simulink model "Dynamics_2024"  (R2024b)
settings: Solver=FixedStepAuto  StartTime=0  StopTime=268704.3823  FixedStep=10  RelTol=1e-12  AbsTol=1e-12
values from neighbouring files (symbols this model uses):
  Disturbances = 1    [Main.m]
  kd = 1e-3    (= 0.001)    [Main.m]
  ki = 1e-3    (= 0.001)    [Main.m]
  kp = 2    [Main.m]
  q0 = [  -0.197305854517669 ... (first row only)    [Main.m]
undefined symbols (not defined in the file or in its folder): control, epsilon, Fe_sun, G, Ix, Iy, Iz, J_e, magnitude, mt, mu_e, mu_sun, r_0ts, R_e, Satellite, v0, v_0ts, w_0, w_desired, x0
libraries: matrix_library x2, vrlib x1
settings Model: Creator=marty  LastModifiedBy=marty

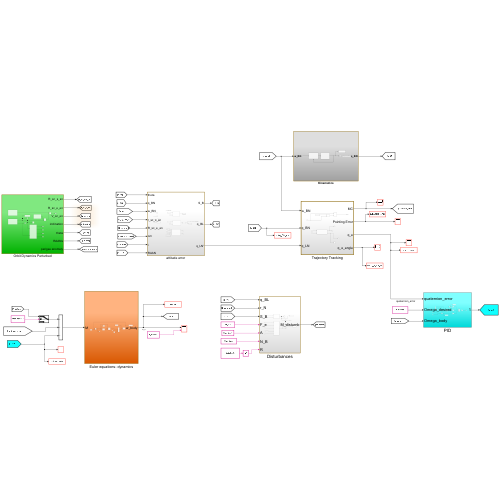
[thumbnail: Simulink's stored preview of the top-level diagram]
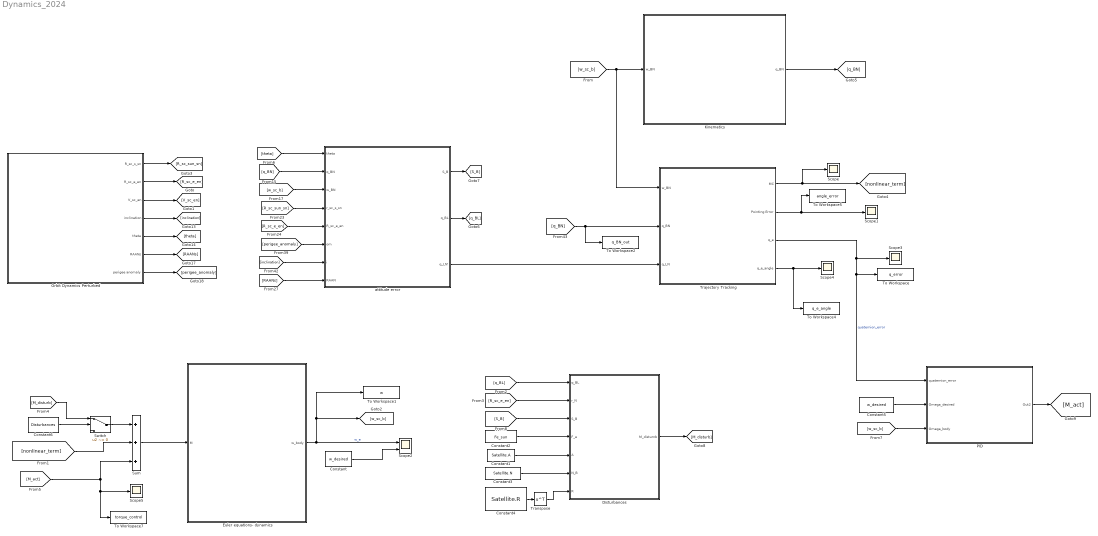
== system Dynamics_2024 ==
  Constant : Constant  Value=w_desired
  Constant1 : Constant  Value=Satellite.A
  Constant2 : Constant  Value=Fe_sun
  Constant3 : Constant  Value=Satellite.N
  Constant4 : Constant  Value=Satellite.R
  Constant5 : Constant  Value=w_desired
  Constant6 : Constant  Value=Disturbances
  Disturbances : Subsystem
  Euler equations- dynamics : Subsystem
  Kinematics : Subsystem
  Orbit Dynamics Perturbed : Subsystem
  PID : Subsystem
  Scope{,1,3..5} (5 alike) : Scope
  Scope2 : Scope  NumInputPorts=2
  Sum : Sum  Inputs=+++
  Switch : Switch  Criteria=u2 ~= 0  SaturateOnIntegerOverflow=off  InputSameDT=off
  To Workspace : ToWorkspace  VariableName=q_error  SampleTime=-1
  To Workspace1 : ToWorkspace  VariableName=w  SampleTime=-1
  To Workspace2 : ToWorkspace  VariableName=q_BN_out  SampleTime=-1
  To Workspace4 : ToWorkspace  VariableName=q_e_angle  SampleTime=-1
  To Workspace5 : ToWorkspace  VariableName=angle_error  SampleTime=-1
  To Workspace7 : ToWorkspace  VariableName=torque_control  SampleTime=-1
  Trajectory Tracking : Subsystem  TreatAsAtomicUnit=on
  Transpose : Math  Operator=transpose
  attitude error : Subsystem
  wires:
  attitude error/2(q_BL) -> [q_BL]
  [R_sc_e_en] -> attitude error/5(R_sc_e_en)
  Orbit Dynamics Perturbed/7(perigee anomaly) -> [perigee_anomaly]
  Constant/1 -> Scope2/2
  [inclination] -> attitude error/7(i)
  [R_sc_sun_sn] -> attitude error/4(r_sc_s_sn)
  Trajectory Tracking/2(Pointing Error) -> To Workspace5/1, Scope1/1
  attitude error/3(q_LN') -> Trajectory Tracking/3(q_LN)
  Orbit Dynamics Perturbed/1(R_sc_s_sn) -> [R_sc_sun_sn]
  Orbit Dynamics Perturbed/2(R_sc_e_en) -> [R_sc_e_en]
  Orbit Dynamics Perturbed/4(inclination) -> [inclination]
  [w_sc_b] -> attitude error/3(w_BN)
  [w_sc_b] -> Kinematics/1(w_BN), Trajectory Tracking/1(w_BN)
  [perigee_anomaly] -> attitude error/6(om)
  Orbit Dynamics Perturbed/3(V_sc_en) -> [V_sc_en]
  Orbit Dynamics Perturbed/6(RAANs) -> [RAANs]
  Sum/1 -> Euler equations- dynamics/1(M)
  [RAANs] -> attitude error/8(RAAN)
  [q_BN] -> attitude error/2(q_BN)
  attitude error/1(S_B) -> [S_B]
  Kinematics/1(q_BN) -> [q_BN]
  Orbit Dynamics Perturbed/5(theta) -> [theta]
  [theta] -> attitude error/1(theta)
  [q_BN] -> To Workspace2/1, Trajectory Tracking/2(q_BN)
  Constant4/1 -> Transpose/1
  [q_BL] -> Disturbances/1(q_BL)
  [R_sc_e_en] -> Disturbances/2(r_N)
  [S_B] -> Disturbances/3(S_B)
  Constant2/1 -> Disturbances/4(F_e)
  Constant1/1 -> Disturbances/5(A)
  Constant3/1 -> Disturbances/6(N_B)
  Transpose/1 -> Disturbances/7(R)
  Disturbances/1(M_disturnb) -> [M_disturb]
  [M_disturb] -> Switch/1
  Trajectory Tracking/4(q_e_angle) -> To Workspace4/1, Scope4/1
  Euler equations- dynamics/1(w_body) -> To Workspace1/1, [w_sc_b], Scope2/1  "w_e"
  Trajectory Tracking/3(q_e) -> PID/1(quaternion_error), To Workspace/1, Scope3/1  "quaternion_error"
  Trajectory Tracking/1(MC) -> Scope/1, [nonlinear_term]
  [nonlinear_term] -> Sum/2
  Switch/1 -> Sum/1
  Constant6/1 -> Switch/2
  [M_act] -> Sum/3, Scope5/1, To Workspace7/1
  Constant5/1 -> PID/2(Omega_desired)
  [w_sc_b] -> PID/3(Omega_body)
  PID/1(Out2) -> [M_act]

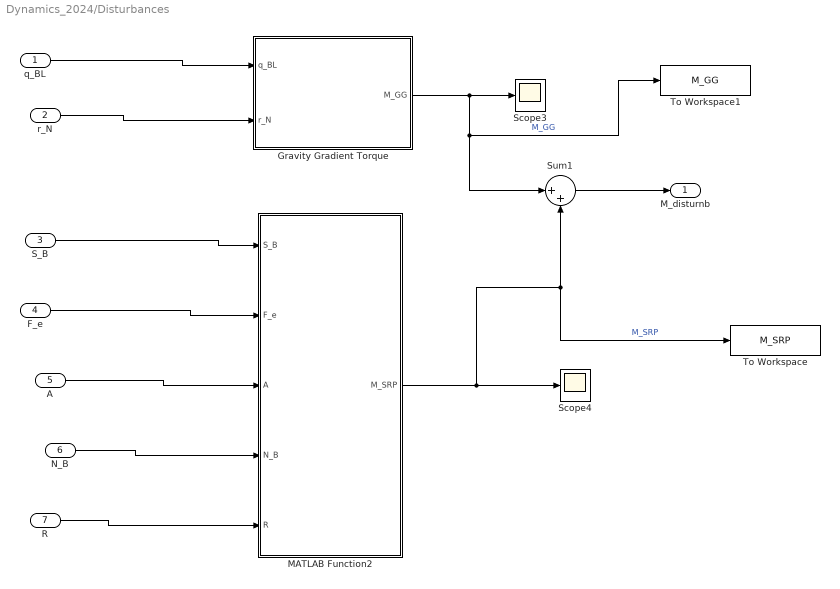
== system Dynamics_2024/Disturbances ==
  q_BL : Inport
  r_N : Inport  Port=2
  S_B : Inport  Port=3
  F_e : Inport  Port=4
  A : Inport  Port=5
  N_B : Inport  Port=6
  R : Inport  Port=7
  Gravity Gradient Torque : Subsystem
  MATLAB Function2 : MATLAB Function  TreatAsAtomicUnit=on
  Scope3 : Scope
  Scope4 : Scope
  Sum1 : Sum  Inputs=|++
  To Workspace : ToWorkspace  VariableName=M_SRP  SampleTime=-1
  To Workspace1 : ToWorkspace  VariableName=M_GG  SampleTime=-1
  M_disturnb : Outport
  wires:
  R/1 -> MATLAB Function2/5(R)
  MATLAB Function2/1(M_SRP) -> Sum1/2, To Workspace/1, Scope4/1  "M_SRP"
  F_e/1 -> MATLAB Function2/2(F_e)
  Gravity Gradient Torque/1(M_GG) -> To Workspace1/1, Sum1/1, Scope3/1  "M_GG"
  q_BL/1 -> Gravity Gradient Torque/1(q_BL)
  r_N/1 -> Gravity Gradient Torque/2(r_N)
  N_B/1 -> MATLAB Function2/4(N_B)
  A/1 -> MATLAB Function2/3(A)
  S_B/1 -> MATLAB Function2/1(S_B)
  Sum1/1 -> M_disturnb/1

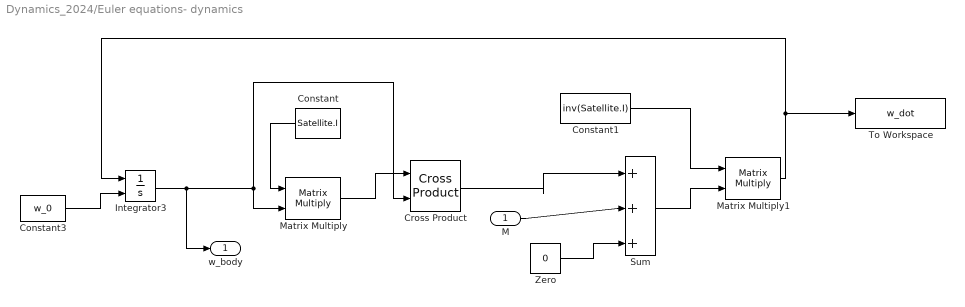
== system Dynamics_2024/Euler equations- dynamics ==
  M : Inport
  Constant : Constant  Value=Satellite.I
  Constant1 : Constant  Value=inv(Satellite.I)
  Constant3 : Constant  Value=w_0
  Cross Product : matrix_library/Cross Product
  Integrator3 : Integrator  InitialConditionSource=external
  Matrix Multiply : Product  Multiplication=Matrix(*)
  Matrix Multiply1 : Product  Multiplication=Matrix(*)
  Sum : Sum  Inputs=|+++
  To Workspace : ToWorkspace  VariableName=w_dot  SampleTime=-1
  Zero : Constant  Value=0  OutDataTypeStr=Inherit: Inherit via back propagation
  w_body : Outport
  wires:
  Constant3/1 -> Integrator3/2
  Integrator3/1 -> w_body/1, Matrix Multiply/2, Cross Product/2
  Matrix Multiply/1 -> Cross Product/1
  Constant1/1 -> Matrix Multiply1/1
  Matrix Multiply1/1 -> Integrator3/1, To Workspace/1
  Constant/1 -> Matrix Multiply/1
  Cross Product/1 -> Sum/1
  Sum/1 -> Matrix Multiply1/2
  M/1 -> Sum/2
  Zero/1 -> Sum/3

== system Dynamics_2024/Kinematics ==
  note: (Body Frame Quaternion)
  w_BN : Inport
  Quaternion Normalisation : Subsystem
  Quaternions : Subsystem
      settings: PortSchema="{\"entries\":[{\"content\":{\"sides\":[{\"content\":{\"connectorIds\":[\"In1\"]},\"type\":\"ConnectorPlacement.EquallySpacedRectSide\",\"uuid\":\"337480c7-b996-434a-97d1-93b75d8b293c\"},{\"content\":{\"connectorIds\":[\"Out1\"],\"side\":\"RIGHT\"},\"type\":\"ConnectorPlacement.EquallySpacedRectSide\",\"uuid\":\"41d32615-4344-48a4-ad5b-2dad4deabdda\"},{\"content\":{\"side\":\"TOP\"},\"type\":\"ConnectorPlacement.EquallySpacedRectSide\",\"uuid\":\"47835596-097d-48d1-90ae-77b48fddf76d\"},{\"content\":{\"connectorIds\":[\"In2\"],\"side\":\"BOTTOM\"},\"type\":\"ConnectorPlacement.EquallySpacedRectSide\",\"uuid\":\"9f38fa4d-c6c1-4321-9750-02b4f73c744f\"}]},\"type\":\"ConnectorPlacement.EquallySpacedConnector\",\"uuid\":\"8ea16f6d-57f4-43cd-ae9c-44a64026dd8f\"}],\"packageUris\":[\"http://schema.mathworks.com/mf0/Connector/R2020b\"],\"version\":\"1.0\"}"
  To Workspace : ToWorkspace  VariableName=q_BN  SampleTime=-1
  q_BN : Outport
  wires:
  w_BN/1 -> Quaternions/1(w)
  Quaternion Normalisation/1(q_BN) -> To Workspace/1, q_BN/1, Quaternions/2(q_BN)
  Quaternions/1(q(t)) -> Quaternion Normalisation/1(q(t))

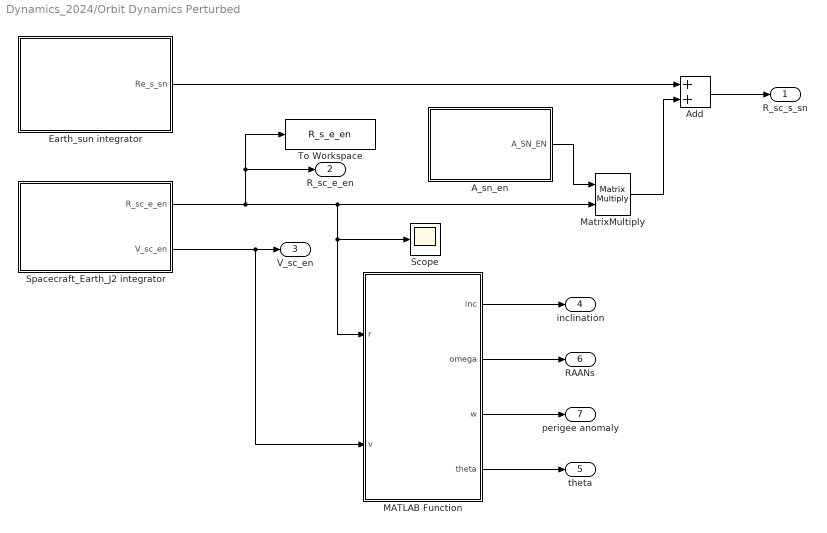
== system Dynamics_2024/Orbit Dynamics Perturbed ==
  A_sn_en : Subsystem
  Add : Sum
  Earth_sun integrator : Subsystem
  MATLAB Function : MATLAB Function  TreatAsAtomicUnit=on
  MatrixMultiply : Product  Multiplication=Matrix(*)
  Scope : Scope
  "Spacecraft_Earth_J2 integrator " : Subsystem
  To Workspace : ToWorkspace  VariableName=R_s_e_en  SampleTime=-1
  R_sc_s_sn : Outport
  R_sc_e_en : Outport  Port=2
  V_sc_en : Outport  Port=3
  inclination : Outport  Port=4
  theta : Outport  Port=5
  RAANs : Outport  Port=6
  perigee anomaly : Outport  Port=7
  wires:
  MatrixMultiply/1 -> Add/2
  A_sn_en/1(A_SN_EN) -> MatrixMultiply/1
  "Spacecraft_Earth_J2 integrator "/2(V_sc_en) -> MATLAB Function/2(v), V_sc_en/1
  "Spacecraft_Earth_J2 integrator "/1(R_sc_e_en) -> R_sc_e_en/1, To Workspace/1, Scope/1, MATLAB Function/1(r), MatrixMultiply/2
  Earth_sun integrator/1(Re_s_sn) -> Add/1
  Add/1 -> R_sc_s_sn/1
  MATLAB Function/1(inc) -> inclination/1
  MATLAB Function/4(theta) -> theta/1
  MATLAB Function/2(omega) -> RAANs/1
  MATLAB Function/3(w) -> perigee anomaly/1

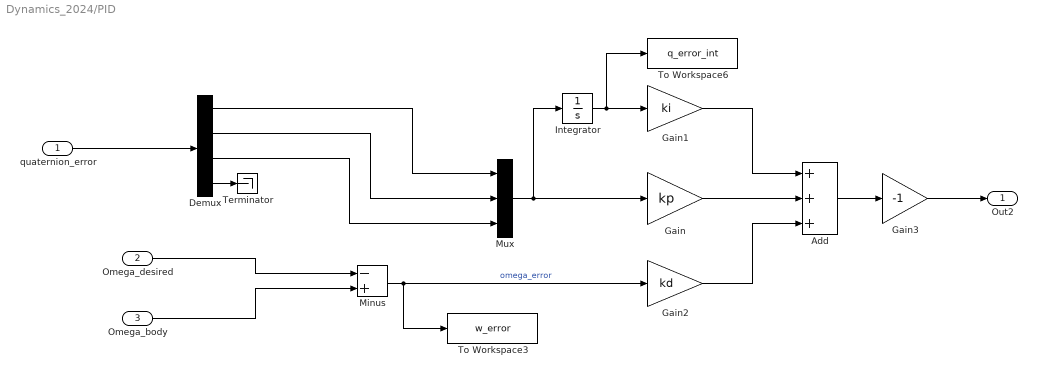
== system Dynamics_2024/PID ==
  quaternion_error : Inport
  Omega_desired : Inport  Port=2
  Omega_body : Inport  Port=3
  Add : Sum  Inputs=+++
  Demux : Demux
  Gain : Gain  Gain=kp
  Gain1 : Gain  Gain=ki
  Gain2 : Gain  Gain=kd
  Gain3 : Gain  Gain=-1
  Integrator : Integrator
  Minus : Sum  Inputs=-+
  Mux : Mux  Inputs=3
  Terminator : Terminator
  To Workspace3 : ToWorkspace  VariableName=w_error  SampleTime=-1
  To Workspace6 : ToWorkspace  VariableName=q_error_int  SampleTime=-1
  Out2 : Outport
  wires:
  Minus/1 -> To Workspace3/1, Gain2/1  "omega_error"
  Integrator/1 -> To Workspace6/1, Gain1/1
  Add/1 -> Gain3/1
  Demux/2 -> Mux/2
  Demux/3 -> Mux/3
  Gain1/1 -> Add/1
  Omega_desired/1 -> Minus/1
  Demux/1 -> Mux/1
  Gain2/1 -> Add/3
  Mux/1 -> Integrator/1, Gain/1
  Gain/1 -> Add/2
  Demux/4 -> Terminator/1
  Omega_body/1 -> Minus/2
  Gain3/1 -> Out2/1
  quaternion_error/1 -> Demux/1

== system Dynamics_2024/Trajectory Tracking ==
  note: ref
  w_BN : Inport
  q_BN : Inport  Port=2
  q_LN : Inport  Port=3
  Constant2 : Constant  Value=Satellite.I
  Cross Product : matrix_library/Cross Product
  Pointing Error for Slew Maneuvre : Subsystem
  Product1 : Product  Multiplication=Matrix(*)
  Scope : Scope
  MC : Outport
  Pointing Error : Outport  Port=2
  q_e : Outport  Port=3
  q_e_angle : Outport  Port=4
  wires:
  q_BN/1 -> Pointing Error for Slew Maneuvre/2(q_Est)  "q_BN"
  Product1/1 -> Cross Product/2
  Constant2/1 -> Product1/1
  Cross Product/1 -> MC/1
  w_BN/1 -> Product1/2, Cross Product/1
  q_LN/1 -> Pointing Error for Slew Maneuvre/1(q_LN)
  Pointing Error for Slew Maneuvre/1(Pointing Error) -> q_e_angle/1, Pointing Error/1  "pointing error"
  Pointing Error for Slew Maneuvre/2(q_e) -> Scope/1, q_e/1  "q_e"

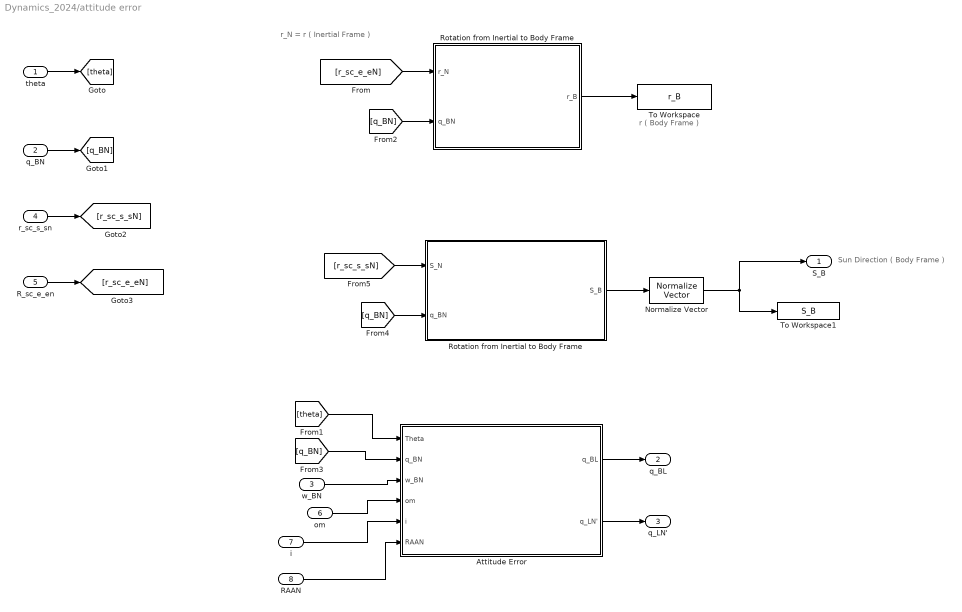
== system Dynamics_2024/attitude error ==
  note: r_N = r ( Inertial Frame )
  note: Sun Direction ( Body Frame )
  note: r ( Body Frame )
  theta : Inport
  q_BN : Inport  Port=2
  w_BN : Inport  Port=3
  r_sc_s_sn : Inport  Port=4
  R_sc_e_en : Inport  Port=5
  om : Inport  Port=6
  i : Inport  Port=7
  RAAN : Inport  Port=8
  " Rotation from Inertial to Body Frame" : Subsystem
  Attitude Error : Subsystem
  Normalize Vector : vrlib/Utilities/Normalize Vector  maxzero=0
  Rotation from Inertial to Body Frame : Subsystem
  To Workspace : ToWorkspace  VariableName=r_B  SampleTime=-1
  To Workspace1 : ToWorkspace  VariableName=S_B  SampleTime=-1
  S_B : Outport
  q_BL : Outport  Port=2
  q_LN' : Outport  Port=3
  wires:
  Normalize Vector/1 -> S_B/1, To Workspace1/1
  w_BN/1 -> Attitude Error/3(w_BN)
  Rotation from Inertial to Body Frame/1(S_B) -> Normalize Vector/1
  " Rotation from Inertial to Body Frame"/1(r_B) -> To Workspace/1
  Attitude Error/1(q_BL) -> q_BL/1
  Attitude Error/2(q_LN') -> q_LN'/1
  theta/1 -> [theta]
  [theta] -> Attitude Error/1(Theta)
  q_BN/1 -> [q_BN]
  [q_BN] -> " Rotation from Inertial to Body Frame"/2(q_BN)
  [q_BN] -> Attitude Error/2(q_BN)
  [q_BN] -> Rotation from Inertial to Body Frame/2(q_BN)
  r_sc_s_sn/1 -> [r_sc_s_sN]
  [r_sc_e_eN] -> " Rotation from Inertial to Body Frame"/1(r_N)
  R_sc_e_en/1 -> [r_sc_e_eN]
  [r_sc_s_sN] -> Rotation from Inertial to Body Frame/1(S_N)
  om/1 -> Attitude Error/4(om)
  i/1 -> Attitude Error/5(i)
  RAAN/1 -> Attitude Error/6(RAAN)

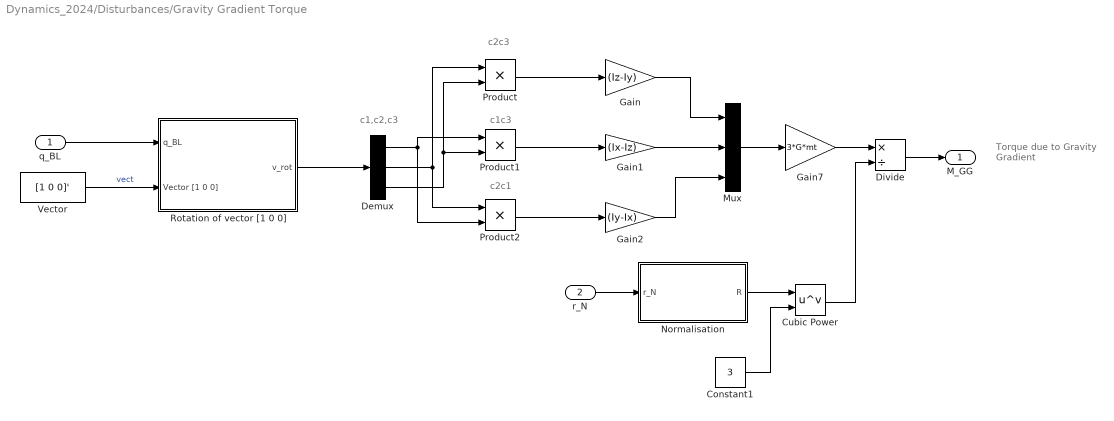
== system Dynamics_2024/Disturbances/Gravity Gradient Torque ==
  note: Torque due to
      | Gravity Gradient
  note: c1c3
  note: c2c3
  note: c2c1
  note: c1,c2,c3
  q_BL : Inport
  r_N : Inport  Port=2
  Constant1 : Constant  Value=3
  Cubic Power : Math  Operator=pow
  Demux : Demux  Outputs=3
  Divide : Product  Inputs=*/
  Gain : Gain  Gain=(Iz-Iy)
  Gain1 : Gain  Gain=(Ix-Iz)
  Gain2 : Gain  Gain=(Iy-Ix)
  Gain7 : Gain  Gain=3*G*mt
  Mux : Mux  Inputs=3
  Normalisation : Subsystem
  Product : Product
  Product1 : Product
  Product2 : Product
  Rotation of vector [1 0 0] : Subsystem
  Vector : Constant  Value=[1 0 0]'
  M_GG : Outport
  wires:
  Cubic Power/1 -> Divide/2
  Demux/1 -> Product1/1, Product2/2
  q_BL/1 -> Rotation of vector [1 0 0]/1(q_BL)
  Rotation of vector [1 0 0]/1(v_rot) -> Demux/1
  Normalisation/1(R) -> Cubic Power/1
  Divide/1 -> M_GG/1
  Vector/1 -> Rotation of vector [1 0 0]/2(Vector [1 0 0])  "vect"
  Product2/1 -> Gain2/1
  Demux/2 -> Product/1, Product2/1
  Mux/1 -> Gain7/1
  r_N/1 -> Normalisation/1(r_N)
  Gain7/1 -> Divide/1
  Demux/3 -> Product1/2, Product/2
  Constant1/1 -> Cubic Power/2
  Gain/1 -> Mux/1
  Gain1/1 -> Mux/2
  Gain2/1 -> Mux/3
  Product1/1 -> Gain1/1
  Product/1 -> Gain/1

== system Dynamics_2024/Kinematics/Quaternion Normalisation ==
  q(t) : Inport
  Divide : Product  Inputs=*/
  Dot Product : DotProduct  OutDataTypeStr=Inherit: Inherit via internal rule
  Sqrt : Sqrt
  q_BN : Outport
  wires:
  Dot Product/1 -> Sqrt/1
  q(t)/1 -> Divide/1, Dot Product/1, Dot Product/2
  Sqrt/1 -> Divide/2
  Divide/1 -> q_BN/1

== system Dynamics_2024/Kinematics/Quaternions ==
  note: Normalised
      | quaternion
  w : Inport
  q_BN : Inport  Port=2
  Gain : Gain  Gain=1/2
  Initial Condition : Constant  Value=q0
  Integrator : Integrator  InitialConditionSource=external
  Matrix Multiply : Product  Multiplication=Matrix(*)
  OMEGA Matrix : Subsystem
  q(t) : Outport
  wires:
  Integrator/1 -> q(t)/1
  Initial Condition/1 -> Integrator/2
  Matrix Multiply/1 -> Integrator/1
  Gain/1 -> Matrix Multiply/1
  w/1 -> OMEGA Matrix/1(w)
  OMEGA Matrix/1(OM Matrix) -> Gain/1
  q_BN/1 -> Matrix Multiply/2

== system Dynamics_2024/Orbit Dynamics Perturbed/A_sn_en ==
  Constant : Constant  Value=epsilon
  Constant1 : Constant
  Gain : Gain  Gain=-1
  Matrix Concatenate : Concatenate  NumInputs=3  Mode=Multidimensional array  ConcatenateDimension=2
  Mux : Mux  Inputs=3
  Mux1 : Mux  Inputs=3
  Mux2 : Mux  Inputs=3
  Trigonometric Function : Trigonometry
  Trigonometric Function1 : Trigonometry  Operator=cos
  Zero : Constant  Value=0  OutDataTypeStr=Inherit: Inherit via back propagation
  A_SN_EN : Outport
  wires:
  Gain/1 -> Mux2/3
  Constant/1 -> Trigonometric Function/1, Trigonometric Function1/1
  Trigonometric Function/1 -> Mux1/2, Gain/1
  Trigonometric Function1/1 -> Mux2/2, Mux1/3
  Constant1/1 -> Mux/1
  Mux1/1 -> Matrix Concatenate/3
  Mux/1 -> Matrix Concatenate/1
  Matrix Concatenate/1 -> A_SN_EN/1
  Mux2/1 -> Matrix Concatenate/2
  Zero/1 -> Mux/2, Mux/3, Mux2/1, Mux1/1

== system Dynamics_2024/Orbit Dynamics Perturbed/Earth_sun integrator ==
  Constant1 : Constant  Value=v_0ts
  Constant3 : Constant  Value=r_0ts
  Constant5 : Constant  Value=3
  Divide : Product  Inputs=*/
  Gain : Gain  Gain=-mu_sun
  Integrator : Integrator  InitialConditionSource=external
  Integrator1 : Integrator  InitialConditionSource=external
  Power : Math  Operator=pow
  norm : Subsystem
  Re_s_sn : Outport
  wires:
  Constant1/1 -> Integrator/2
  Constant3/1 -> Integrator1/2
  Integrator1/1 -> norm/1(vector), Divide/1, Re_s_sn/1
  Gain/1 -> Integrator/1
  Power/1 -> Divide/2
  norm/1(norm(vector)) -> Power/1
  Constant5/1 -> Power/2
  Integrator/1 -> Integrator1/1
  Divide/1 -> Gain/1

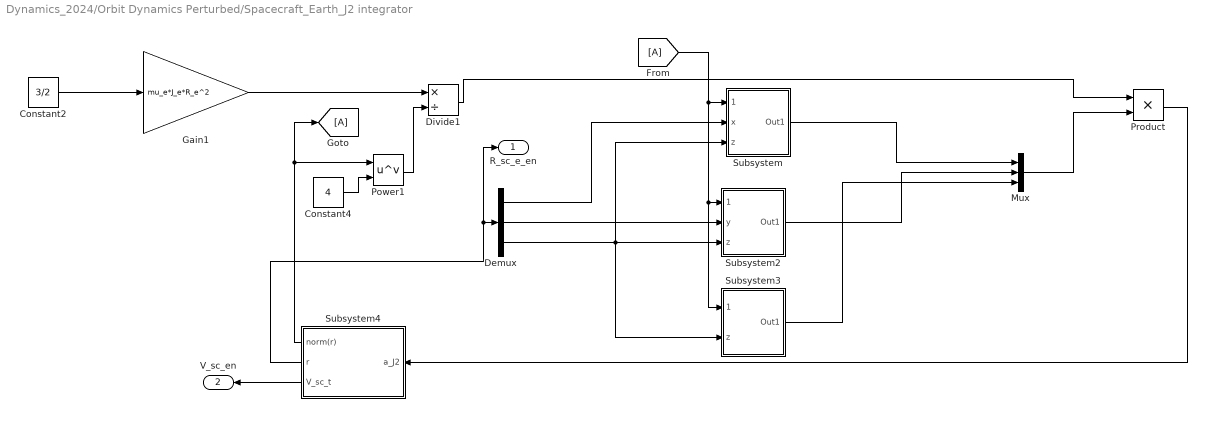
== system Dynamics_2024/Orbit Dynamics Perturbed/Spacecraft_Earth_J2 integrator  ==
  Constant2 : Constant  Value=3/2
  Constant4 : Constant  Value=4
  Demux : Demux  Outputs=3
  Divide1 : Product  Inputs=*/
  From : From
  Gain1 : Gain  Gain=mu_e*J_e*R_e^2
  Goto : Goto
  Mux : Mux  Inputs=3
  Power1 : Math  Operator=pow
  Product : Product
  Subsystem : Subsystem
  Subsystem2 : Subsystem
  Subsystem3 : Subsystem
  Subsystem4 : Subsystem
  R_sc_e_en : Outport
  V_sc_en : Outport  Port=2
  wires:
  Subsystem4/3(V_sc_t) -> V_sc_en/1
  Subsystem4/1(norm(r)) -> Power1/1, Goto/1
  Constant4/1 -> Power1/2
  Demux/2 -> Subsystem2/2(y)
  Divide1/1 -> Product/1
  From/1 -> Subsystem/1(norm(r)), Subsystem2/1(norm(r)), Subsystem3/1(norm(r))
  Demux/3 -> Subsystem3/2(z), Subsystem/3(z), Subsystem2/3(z)
  Constant2/1 -> Gain1/1
  Subsystem3/1(Out1) -> Mux/3
  Subsystem2/1(Out1) -> Mux/2
  Subsystem/1(Out1) -> Mux/1
  Product/1 -> Subsystem4/1(a_J2)
  Demux/1 -> Subsystem/2(x)
  Power1/1 -> Divide1/2
  Gain1/1 -> Divide1/1
  Subsystem4/2(r) -> Demux/1, R_sc_e_en/1
  Mux/1 -> Product/2

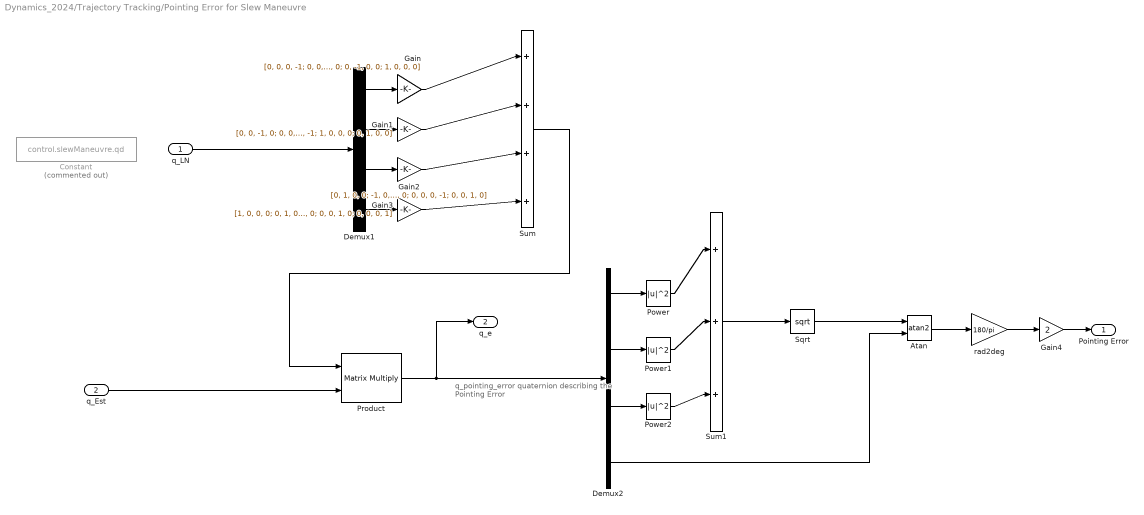
== system Dynamics_2024/Trajectory Tracking/Pointing Error for Slew Maneuvre ==
  note: q_pointing_error
      | quaternion describing the Pointing Error
  q_LN : Inport
  q_Est : Inport  Port=2
  Atan : Trigonometry  Operator=atan2  OutputSignalType=real
  Constant : Constant  Commented=on  Value=control.slewManeuvre.qd
  Demux1 : Demux
  Demux2 : Demux
  Gain : Gain  Gain=[0, 0, 0, -1; 0, 0, 1, 0; 0, -1, 0, 0; 1, 0, 0, 0]
  Gain1 : Gain  Gain=[0, 0, -1, 0; 0, 0, 0, -1; 1, 0, 0, 0; 0, 1, 0, 0]
  Gain2 : Gain  Gain=[0, 1, 0, 0; -1, 0, 0, 0; 0, 0, 0, -1; 0, 0, 1, 0]
  Gain3 : Gain  Gain=[1, 0, 0, 0; 0, 1, 0, 0; 0, 0, 1, 0; 0, 0, 0, 1]
  Gain4 : Gain  Gain=2
  Power : Math  Operator=magnitude^2
  Power1 : Math  Operator=magnitude^2
  Power2 : Math  Operator=magnitude^2
  Product : Product  Multiplication=Matrix(*)
  Sqrt : Sqrt
  Sum : Sum  Inputs=|++++
  Sum1 : Sum  Inputs=|+++
  rad2deg : Gain  Gain=180/pi
  Pointing Error : Outport
  q_e : Outport  Port=2
  wires:
  Power1/1 -> Sum1/2
  Demux2/4 -> Atan/2
  Atan/1 -> rad2deg/1
  Power/1 -> Sum1/1
  Demux2/2 -> Power1/1
  Demux2/3 -> Power2/1
  Demux2/1 -> Power/1
  Sum1/1 -> Sqrt/1
  Power2/1 -> Sum1/3
  Sqrt/1 -> Atan/1
  Product/1 -> Demux2/1, q_e/1
  Gain/1 -> Sum/1
  Gain2/1 -> Sum/3
  Gain1/1 -> Sum/2
  Demux1/3 -> Gain2/1
  Demux1/1 -> Gain/1
  Gain3/1 -> Sum/4
  Demux1/2 -> Gain1/1
  Demux1/4 -> Gain3/1
  Sum/1 -> Product/1
  rad2deg/1 -> Gain4/1
  q_LN/1 -> Demux1/1
  Gain4/1 -> Pointing Error/1
  q_Est/1 -> Product/2

== system Dynamics_2024/attitude error/ Rotation from Inertial to Body Frame ==
  note: Quaternion Rotation (Double Tensor Product)
  note: $r_B = q_{BN}\cdot r_N$
  r_N : Inport
  q_BN : Inport  Port=2
  Demux : Demux
  Mux : Mux  Inputs=3
  Quaternion multiplication 1 : Subsystem
  Quaternion multiplication 2 : Subsystem
  Transformation in Quaternion : Subsystem
  Transpose : Gain  Gain=[-1 -1 -1 1]
  r_B : Outport
  wires:
  r_N/1 -> Transformation in Quaternion/1(r_N)
  Mux/1 -> r_B/1
  Transpose/1 -> Quaternion multiplication 1/1(q_BN (T) = q)
  q_BN/1 -> Quaternion multiplication 2/2(q_BN = q'), Transpose/1
  Transformation in Quaternion/1(q(r_N)) -> Quaternion multiplication 1/2(q(r_N) = q')
  Quaternion multiplication 2/1(q*q' = q2) -> Demux/1
  Quaternion multiplication 1/1(q*q' = q1) -> Quaternion multiplication 2/1(q1 = q)
  Demux/1 -> Mux/1
  Demux/2 -> Mux/2
  Demux/3 -> Mux/3

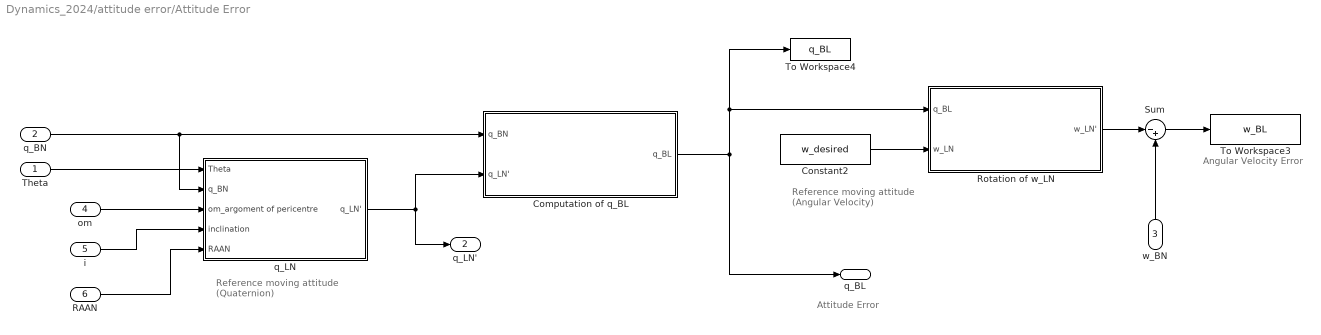
== system Dynamics_2024/attitude error/Attitude Error ==
  note: Angular Velocity Error
  note: Reference moving attitude
      | (Angular Velocity)
  note: Attitude Error
  note: Reference moving attitude
      | (Quaternion)
  Theta : Inport
  q_BN : Inport  Port=2
  w_BN : Inport  Port=3
  om : Inport  Port=4
  i : Inport  Port=5
  RAAN : Inport  Port=6
  Computation of q_BL : Subsystem
  Constant2 : Constant  Value=w_desired
  Rotation of w_LN : Subsystem
  Sum : Sum  Inputs=|-+
  To Workspace3 : ToWorkspace  VariableName=w_BL  SampleTime=-1
  To Workspace4 : ToWorkspace  VariableName=q_BL  SampleTime=-1
  q_LN : Subsystem
  q_BL : Outport
  q_LN' : Outport  Port=2
  wires:
  Computation of q_BL/1(q_BL) -> Rotation of w_LN/1(q_BL), To Workspace4/1, q_BL/1
  Theta/1 -> q_LN/1(Theta)
  Sum/1 -> To Workspace3/1
  Rotation of w_LN/1(w_LN') -> Sum/1
  Constant2/1 -> Rotation of w_LN/2(w_LN)
  q_BN/1 -> q_LN/2(q_BN), Computation of q_BL/1(q_BN)
  q_LN/1(q_LN') -> Computation of q_BL/2(q_LN'), q_LN'/1
  w_BN/1 -> Sum/2
  om/1 -> q_LN/3(om_argoment of pericentre)
  i/1 -> q_LN/4(inclination)
  RAAN/1 -> q_LN/5(RAAN)

== system Dynamics_2024/attitude error/Rotation from Inertial to Body Frame ==
  note: $S_B = q_{BN}\cdot S_N$
  note: Quaternion Rotation (Double Tensor Product)
  S_N : Inport
  q_BN : Inport  Port=2
  Demux : Demux
  Mux : Mux  Inputs=3
  Quaternion multiplication 1 : Subsystem
  Quaternion multiplication 2 : Subsystem
  Transformation in Quaternion : Subsystem
  Transpose : Gain  Gain=[-1 -1 -1 1]
  S_B : Outport
  wires:
  S_N/1 -> Transformation in Quaternion/1(S_N)
  Mux/1 -> S_B/1
  Transpose/1 -> Quaternion multiplication 1/1(q_BN (T) = q)
  q_BN/1 -> Quaternion multiplication 2/2(q_BN = q'), Transpose/1
  Transformation in Quaternion/1(q(S_N)) -> Quaternion multiplication 1/2(q(S_N) = q')
  Quaternion multiplication 2/1(q*q' = q2) -> Demux/1
  Quaternion multiplication 1/1(q*q' = q1) -> Quaternion multiplication 2/1(q1 = q)
  Demux/1 -> Mux/1
  Demux/2 -> Mux/2
  Demux/3 -> Mux/3

== system Dynamics_2024/Disturbances/Gravity Gradient Torque/Normalisation ==
  r_N : Inport
  Dot Product : DotProduct  OutDataTypeStr=Inherit: Inherit via internal rule
  Sqrt : Sqrt
  R : Outport
  wires:
  Dot Product/1 -> Sqrt/1
  r_N/1 -> Dot Product/1, Dot Product/2
  Sqrt/1 -> R/1

== system Dynamics_2024/Disturbances/Gravity Gradient Torque/Rotation of vector [1 0 0] ==
  note: Quaternion Rotation (Double Tensor Product)
  q_BL : Inport
  Vector [1 0 0] : Inport  Port=2
  Demux : Demux
  Mux : Mux  Inputs=3
  Quaternion multiplication 1 : Subsystem
  Quaternion multiplication 2 : Subsystem
  Transformation in Quaternion : Subsystem
  Transpose : Gain  Gain=[-1 -1 -1 1]
  v_rot : Outport
  wires:
  Vector [1 0 0]/1 -> Transformation in Quaternion/1(Vector [1 0 0])
  Mux/1 -> v_rot/1
  Transpose/1 -> Quaternion multiplication 1/1(q_BL = q)
  q_BL/1 -> Quaternion multiplication 2/2(q_BL =  q'), Transpose/1
  Transformation in Quaternion/1(q(vect)) -> Quaternion multiplication 1/2(q(vect) = q')
  Quaternion multiplication 2/1(q*q' = q2) -> Demux/1
  Quaternion multiplication 1/1(q*q' = q1) -> Quaternion multiplication 2/1(q1 = q)
  Demux/1 -> Mux/1
  Demux/2 -> Mux/2
  Demux/3 -> Mux/3

== system Dynamics_2024/Kinematics/Quaternions/OMEGA Matrix ==
  note: Angular velocity
      | components
  w : Inport
  Demux : Demux  Outputs=3
  Gain1 : Gain  Gain=[0 0 0 1; 0 0 1 0; 0 -1 0 0; -1 0 0 0]
  Gain2 : Gain  Gain=[0 0 -1 0; 0 0 0 1; 1 0 0 0; 0 -1 0 0]
  Gain3 : Gain  Gain=[0 1 0 0; -1 0 0 0; 0 0 0 1; 0 0 -1 0]
  Sum : Sum  Inputs=+++
  OM Matrix : Outport
  wires:
  w/1 -> Demux/1
  Sum/1 -> OM Matrix/1
  Gain3/1 -> Sum/3
  Gain1/1 -> Sum/1
  Demux/2 -> Gain2/1
  Demux/1 -> Gain1/1
  Gain2/1 -> Sum/2
  Demux/3 -> Gain3/1

== system Dynamics_2024/Orbit Dynamics Perturbed/Earth_sun integrator/norm ==
  vector : Inport
  Dot Product : DotProduct  OutDataTypeStr=Inherit: Inherit via internal rule
  Sqrt : Sqrt
  norm(vector) : Outport
  wires:
  Sqrt/1 -> norm(vector)/1
  Dot Product/1 -> Sqrt/1
  vector/1 -> Dot Product/2, Dot Product/1

== system Dynamics_2024/Orbit Dynamics Perturbed/Spacecraft_Earth_J2 integrator /Subsystem ==
  norm(r) : Inport
  x : Inport  Port=2
  z : Inport  Port=3
  Add : Sum  Inputs=+-
  Constant5 : Constant  Value=2
  Constant6 : Constant
  Divide2 : Product  Inputs=*/
  Divide3 : Product  Inputs=*/
  Gain2 : Gain  Gain=5
  Power2 : Math  Operator=pow
  Product : Product
  Out1 : Outport
  wires:
  Gain2/1 -> Add/1
  Add/1 -> Product/2
  Product/1 -> Out1/1
  Power2/1 -> Gain2/1
  x/1 -> Divide2/1
  Constant6/1 -> Add/2
  z/1 -> Divide3/1
  Divide2/1 -> Product/1
  Divide3/1 -> Power2/1
  norm(r)/1 -> Divide3/2, Divide2/2
  Constant5/1 -> Power2/2

== system Dynamics_2024/Orbit Dynamics Perturbed/Spacecraft_Earth_J2 integrator /Subsystem2 ==
  norm(r) : Inport
  y : Inport  Port=2
  z : Inport  Port=3
  Add : Sum  Inputs=+-
  Constant5 : Constant  Value=2
  Constant6 : Constant
  Divide2 : Product  Inputs=*/
  Divide3 : Product  Inputs=*/
  Gain2 : Gain  Gain=5
  Power2 : Math  Operator=pow
  Product : Product
  Out1 : Outport
  wires:
  Gain2/1 -> Add/1
  Constant6/1 -> Add/2
  Divide2/1 -> Product/1
  Product/1 -> Out1/1
  Add/1 -> Product/2
  Constant5/1 -> Power2/2
  norm(r)/1 -> Divide3/2, Divide2/2
  Divide3/1 -> Power2/1
  z/1 -> Divide3/1
  y/1 -> Divide2/1
  Power2/1 -> Gain2/1

== system Dynamics_2024/Orbit Dynamics Perturbed/Spacecraft_Earth_J2 integrator /Subsystem3 ==
  norm(r) : Inport
  z : Inport  Port=2
  Add : Sum  Inputs=+-
  Constant5 : Constant  Value=2
  Constant6 : Constant  Value=3
  Divide2 : Product  Inputs=*/
  Divide3 : Product  Inputs=*/
  Gain2 : Gain  Gain=5
  Power2 : Math  Operator=pow
  Product : Product
  Out1 : Outport
  wires:
  Gain2/1 -> Add/1
  Constant6/1 -> Add/2
  Divide2/1 -> Product/1
  Product/1 -> Out1/1
  Add/1 -> Product/2
  Power2/1 -> Gain2/1
  z/1 -> Divide2/1, Divide3/1
  Divide3/1 -> Power2/1
  norm(r)/1 -> Divide2/2, Divide3/2
  Constant5/1 -> Power2/2

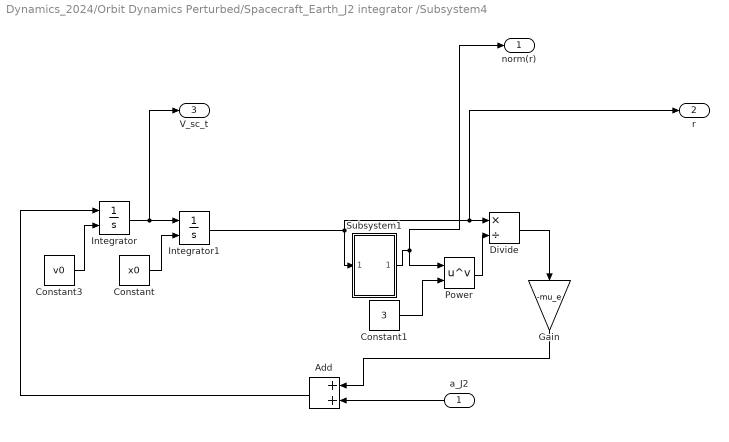
== system Dynamics_2024/Orbit Dynamics Perturbed/Spacecraft_Earth_J2 integrator /Subsystem4 ==
  a_J2 : Inport
  Add : Sum
  Constant : Constant  Value=x0
  Constant1 : Constant  Value=3
  Constant3 : Constant  Value=v0
  Divide : Product  Inputs=*/
  Gain : Gain  Gain=-mu_e
  Integrator : Integrator  InitialConditionSource=external
  Integrator1 : Integrator  InitialConditionSource=external
  Power : Math  Operator=pow
  Subsystem1 : Subsystem
  norm(r) : Outport
  r : Outport  Port=2
  V_sc_t : Outport  Port=3
  wires:
  Constant1/1 -> Power/2
  Gain/1 -> Add/1
  Constant/1 -> Integrator1/2
  Power/1 -> Divide/2
  Divide/1 -> Gain/1
  Integrator1/1 -> Subsystem1/1(In1), Divide/1, r/1
  Integrator/1 -> Integrator1/1, V_sc_t/1
  Add/1 -> Integrator/1
  Subsystem1/1(Out1) -> Power/1, norm(r)/1
  Constant3/1 -> Integrator/2
  a_J2/1 -> Add/2

== system Dynamics_2024/attitude error/ Rotation from Inertial to Body Frame/Quaternion multiplication 1 ==
  q_BN (T) = q : Inport
  q(r_N) = q' : Inport  Port=2
  Demux : Demux
  Gain : Gain  Gain=[1 0 0 0; 0 1 0 0; 0 0 1 0; 0 0 0 1]
  Gain1 : Gain  Gain=[0 0 0 1; 0 0 1 0 ;0 -1 0 0; -1 0 0 0]
  Gain2 : Gain  Gain=[0 0 -1 0; 0 0 0 1; 1 0 0 0; 0 -1 0 0]
  Gain3 : Gain  Gain=[0 1 0 0; -1 0 0 0; 0 0 0 1; 0 0 -1 0]
  Product : Product  Multiplication=Matrix(*)
  Sum : Sum  Inputs=|++++
  q*q' = q1 : Outport
  wires:
  q(r_N) = q'/1 -> Demux/1
  Demux/4 -> Gain/1
  Demux/1 -> Gain1/1
  Demux/2 -> Gain2/1
  Demux/3 -> Gain3/1
  Gain1/1 -> Sum/1
  Gain2/1 -> Sum/2
  Gain3/1 -> Sum/3
  Gain/1 -> Sum/4
  q_BN (T) = q/1 -> Product/2
  Sum/1 -> Product/1
  Product/1 -> q*q' = q1/1

== system Dynamics_2024/attitude error/ Rotation from Inertial to Body Frame/Quaternion multiplication 2 ==
  q1 = q : Inport
  q_BN = q' : Inport  Port=2
  Demux : Demux
  Gain : Gain  Gain=[1 0 0 0;0 1 0 0;0 0 1 0; 0 0 0 1]
  Gain1 : Gain  Gain=[0 0 0 1;0 0 1 0;0 -1 0 0;-1 0 0 0]
  Gain2 : Gain  Gain=[0 0 -1 0;0 0 0 1;1 0 0 0;0 -1 0 0]
  Gain3 : Gain  Gain=[0 1 0 0;-1 0 0 0;0 0 0 1;0 0 -1 0]
  Product : Product  Multiplication=Matrix(*)
  Sum : Sum  Inputs=|++++
  q*q' = q2 : Outport
  wires:
  q_BN = q'/1 -> Demux/1
  Demux/4 -> Gain/1
  Demux/1 -> Gain1/1
  Demux/2 -> Gain2/1
  Demux/3 -> Gain3/1
  Gain1/1 -> Sum/1
  Gain2/1 -> Sum/2
  Gain3/1 -> Sum/3
  Gain/1 -> Sum/4
  q1 = q/1 -> Product/2
  Sum/1 -> Product/1
  Product/1 -> q*q' = q2/1

== system Dynamics_2024/attitude error/ Rotation from Inertial to Body Frame/Transformation in Quaternion ==
  note: Adding 0 as fourth element
      | to match the Quaternion's dimensions
  r_N : Inport
  Constant : Constant  Value=0
  Demux : Demux  Outputs=3
  Mux : Mux
  q(r_N) : Outport
  wires:
  r_N/1 -> Demux/1
  Mux/1 -> q(r_N)/1
  Constant/1 -> Mux/4
  Demux/3 -> Mux/3
  Demux/2 -> Mux/2
  Demux/1 -> Mux/1

== system Dynamics_2024/attitude error/Attitude Error/Computation of q_BL ==
  note: $q_{BL} = q_{LN}'\otimes q_{BN}$
  note: Components of q_LN
  note: Tensor product to compute the error
  q_BN : Inport
  q_LN' : Inport  Port=2
  Demux : Demux
  Gain : Gain  Gain=[0,0,0,-1; 0,0,1,0; 0,-1,0,0; 1,0,0,0]
  Gain1 : Gain  Gain=[0,0,-1,0; 0,0,0,-1; 1,0,0,0; 0,1,0,0]
  Gain2 : Gain  Gain=[0, 1, 0, 0; -1, 0, 0, 0; 0, 0, 0, -1; 0, 0, 1, 0]
  Gain3 : Gain  Gain=[1,0,0,0; 0,1,0,0; 0,0,1,0; 0,0,0,1]
  Product : Product  Multiplication=Matrix(*)
  Sum : Sum  Inputs=|++++
  q_BL : Outport
  wires:
  q_LN'/1 -> Demux/1
  Demux/1 -> Gain/1
  Demux/2 -> Gain1/1
  Demux/3 -> Gain2/1
  Demux/4 -> Gain3/1
  Gain/1 -> Sum/1
  Gain1/1 -> Sum/2
  Gain2/1 -> Sum/3
  Gain3/1 -> Sum/4
  Sum/1 -> Product/1
  q_BN/1 -> Product/2
  Product/1 -> q_BL/1

== system Dynamics_2024/attitude error/Attitude Error/Rotation of w_LN ==
  note: Quaternion Rotation (Double Tensor Product)
  q_BL : Inport
  w_LN : Inport  Port=2
  Demux : Demux
  Mux : Mux  Inputs=3
  Quaternion multiplication 1 : Subsystem
  Quaternion multiplication 2 : Subsystem
  To Workspace : ToWorkspace  VariableName=w_LN_B  SampleTime=-1
  Transformation in Quaternion : Subsystem
  Transpose : Gain  Gain=[-1 -1 -1 1]
  w_LN' : Outport
  wires:
  w_LN/1 -> Transformation in Quaternion/1(w_LN)
  Mux/1 -> To Workspace/1, w_LN'/1
  Transpose/1 -> Quaternion multiplication 1/1(q_BL' = q)
  q_BL/1 -> Quaternion multiplication 2/2(q_BL = q'), Transpose/1
  Transformation in Quaternion/1(q_LN) -> Quaternion multiplication 1/2(q_LN = q')
  Quaternion multiplication 2/1(q*q' = q2) -> Demux/1
  Quaternion multiplication 1/1(q*q' = q1) -> Quaternion multiplication 2/1(q1 = q)
  Demux/1 -> Mux/1
  Demux/2 -> Mux/2
  Demux/3 -> Mux/3

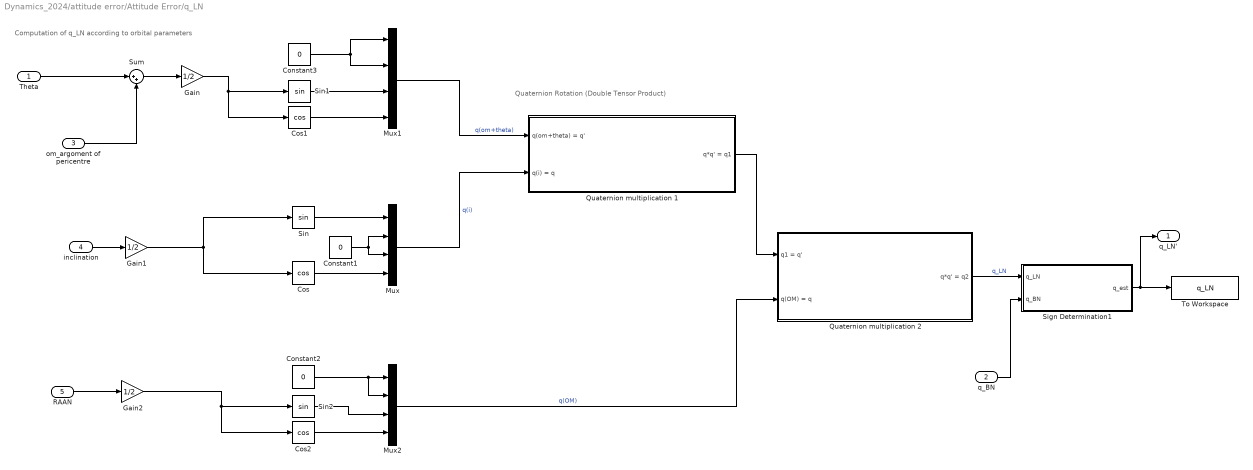
== system Dynamics_2024/attitude error/Attitude Error/q_LN ==
  note: Quaternion Rotation (Double Tensor Product)
  note: Computation of q_LN according to orbital parameters
  Theta : Inport
  q_BN : Inport  Port=2
  om_argoment of pericentre : Inport  Port=3
  inclination : Inport  Port=4
  RAAN : Inport  Port=5
  Constant1 : Constant  Value=0
  Constant2 : Constant  Value=0
  Constant3 : Constant  Value=0
  Cos : Trigonometry  Operator=cos
  Cos1 : Trigonometry  Operator=cos
  Cos2 : Trigonometry  Operator=cos
  Gain : Gain  Gain=1/2
  Gain1 : Gain  Gain=1/2
  Gain2 : Gain  Gain=1/2
  Mux : Mux
  Mux1 : Mux
  Mux2 : Mux
  Quaternion multiplication 1 : Subsystem
  Quaternion multiplication 2 : Subsystem
  Sign Determination1 : Subsystem
  Sin : Trigonometry
  Sin1 : Trigonometry
  Sin2 : Trigonometry
  Sum : Sum  Inputs=|++
  To Workspace : ToWorkspace  VariableName=q_LN  SampleTime=-1
  q_LN' : Outport
  wires:
  Cos/1 -> Mux/4
  Sin/1 -> Mux/1
  Constant1/1 -> Mux/2, Mux/3
  Cos1/1 -> Mux1/4
  Constant3/1 -> Mux1/1, Mux1/2
  Sin1/1 -> Mux1/3
  Gain/1 -> Sin1/1, Cos1/1
  Gain1/1 -> Cos/1, Sin/1
  Theta/1 -> Sum/1
  Cos2/1 -> Mux2/4
  Gain2/1 -> Sin2/1, Cos2/1
  Sin2/1 -> Mux2/3
  Constant2/1 -> Mux2/2, Mux2/1
  om_argoment of pericentre/1 -> Sum/2
  Sum/1 -> Gain/1
  Mux1/1 -> Quaternion multiplication 1/1(q(om+theta) = q')  "q(om+theta)"
  Mux/1 -> Quaternion multiplication 1/2(q(i) = q)  "q(i)"
  Quaternion multiplication 1/1(q*q' = q1) -> Quaternion multiplication 2/1(q1 = q')
  Mux2/1 -> Quaternion multiplication 2/2(q(OM) = q)  "q(OM)"
  Quaternion multiplication 2/1(q*q' = q2) -> Sign Determination1/1("q_LN ")  "q_LN"
  Sign Determination1/1(q_est) -> q_LN'/1, To Workspace/1
  q_BN/1 -> Sign Determination1/2(q_BN)
  inclination/1 -> Gain1/1
  RAAN/1 -> Gain2/1

== system Dynamics_2024/attitude error/Rotation from Inertial to Body Frame/Quaternion multiplication 1 ==
  q_BN (T) = q : Inport
  q(S_N) = q' : Inport  Port=2
  Demux : Demux
  Gain : Gain  Gain=[1 0 0 0; 0 1 0 0; 0 0 1 0; 0 0 0 1]
  Gain1 : Gain  Gain=[0 0 0 1; 0 0 1 0; 0 -1 0 0; -1 0 0 0]
  Gain2 : Gain  Gain=[0 0 -1 0; 0 0 0 1; 1 0 0 0; 0 -1 0 0]
  Gain3 : Gain  Gain=[0 1 0 0; -1 0 0 0; 0 0 0 1; 0 0 -1 0]
  Product : Product  Multiplication=Matrix(*)
  Sum : Sum  Inputs=|++++
  q*q' = q1 : Outport
  wires:
  q(S_N) = q'/1 -> Demux/1
  Demux/4 -> Gain/1
  Demux/1 -> Gain1/1
  Demux/2 -> Gain2/1
  Demux/3 -> Gain3/1
  Gain1/1 -> Sum/1
  Gain2/1 -> Sum/2
  Gain3/1 -> Sum/3
  Gain/1 -> Sum/4
  q_BN (T) = q/1 -> Product/2
  Sum/1 -> Product/1
  Product/1 -> q*q' = q1/1

== system Dynamics_2024/attitude error/Rotation from Inertial to Body Frame/Quaternion multiplication 2 ==
  q1 = q : Inport
  q_BN = q' : Inport  Port=2
  Demux : Demux
  Gain : Gain  Gain=[1 0 0 0; 0 1 0 0; 0 0 1 0; 0 0 0 1]
  Gain1 : Gain  Gain=[0 0 0 1; 0 0 1 0; 0 -1 0 0; -1 0 0 0]
  Gain2 : Gain  Gain=[0 0 -1 0; 0 0 0 1; 1 0 0 0; 0 -1 0 0]
  Gain3 : Gain  Gain=[0 1 0 0; -1 0 0 0; 0 0 0 1; 0 0 -1 0]
  Product : Product  Multiplication=Matrix(*)
  Sum : Sum  Inputs=|++++
  q*q' = q2 : Outport
  wires:
  q_BN = q'/1 -> Demux/1
  Demux/4 -> Gain/1
  Demux/1 -> Gain1/1
  Demux/2 -> Gain2/1
  Demux/3 -> Gain3/1
  Gain1/1 -> Sum/1
  Gain2/1 -> Sum/2
  Gain3/1 -> Sum/3
  Gain/1 -> Sum/4
  q1 = q/1 -> Product/2
  Sum/1 -> Product/1
  Product/1 -> q*q' = q2/1

== system Dynamics_2024/attitude error/Rotation from Inertial to Body Frame/Transformation in Quaternion ==
  note: Adding 0 as fourth element
      | to match the Quaternion's dimensions
  S_N : Inport
  Constant : Constant  Value=0
  Demux : Demux  Outputs=3
  Mux : Mux
  q(S_N) : Outport
  wires:
  S_N/1 -> Demux/1
  Mux/1 -> q(S_N)/1
  Constant/1 -> Mux/4
  Demux/3 -> Mux/3
  Demux/2 -> Mux/2
  Demux/1 -> Mux/1

== system Dynamics_2024/Disturbances/Gravity Gradient Torque/Rotation of vector [1 0 0]/Quaternion multiplication 1 ==
  q_BL = q : Inport
  q(vect) = q' : Inport  Port=2
  Demux : Demux
  Gain : Gain  Gain=[1 0 0 0; 0 1 0 0; 0 0 1 0; 0 0 0 1]
  Gain1 : Gain  Gain=[0 0 0 1; 0 0 1 0; 0 -1 0 0; -1 0 0 0]
  Gain2 : Gain  Gain=[0 0 -1 0; 0 0 0 1; 1 0 0 0; 0 -1 0 0]
  Gain3 : Gain  Gain=[0 1 0 0; -1 0 0 0; 0 0 0 1; 0 0 -1 0]
  Product : Product  Multiplication=Matrix(*)
  Sum : Sum  Inputs=|++++
  q*q' = q1 : Outport
  wires:
  q(vect) = q'/1 -> Demux/1
  Demux/4 -> Gain/1
  Demux/1 -> Gain1/1
  Demux/2 -> Gain2/1
  Demux/3 -> Gain3/1
  Gain1/1 -> Sum/1
  Gain2/1 -> Sum/2
  Gain3/1 -> Sum/3
  Gain/1 -> Sum/4
  q_BL = q/1 -> Product/2
  Sum/1 -> Product/1
  Product/1 -> q*q' = q1/1

== system Dynamics_2024/Disturbances/Gravity Gradient Torque/Rotation of vector [1 0 0]/Quaternion multiplication 2 ==
  q1 = q : Inport
  q_BL =  q' : Inport  Port=2
  Demux : Demux
  Gain : Gain  Gain=[1 0 0 0; 0 1 0 0; 0 0 1 0; 0 0 0 1]
  Gain1 : Gain  Gain=[0 0 0 1; 0 0 1 0; 0 -1 0 0; -1 0 0 0]
  Gain2 : Gain  Gain=[0 0 -1 0; 0 0 0 1; 1 0 0 0; 0 -1 0 0]
  Gain3 : Gain  Gain=[0 1 0 0; -1 0 0 0; 0 0 0 1; 0 0 -1 0]
  Product : Product  Multiplication=Matrix(*)
  Sum : Sum  Inputs=|++++
  q*q' = q2 : Outport
  wires:
  q_BL =  q'/1 -> Demux/1
  Demux/4 -> Gain/1
  Demux/1 -> Gain1/1
  Demux/2 -> Gain2/1
  Demux/3 -> Gain3/1
  Gain1/1 -> Sum/1
  Gain2/1 -> Sum/2
  Gain3/1 -> Sum/3
  Gain/1 -> Sum/4
  q1 = q/1 -> Product/2
  Sum/1 -> Product/1
  Product/1 -> q*q' = q2/1

== system Dynamics_2024/Disturbances/Gravity Gradient Torque/Rotation of vector [1 0 0]/Transformation in Quaternion ==
  note: Adding 0 as fourth element
      | to match the Quaternion's dimensions
  Vector [1 0 0] : Inport
  Constant : Constant  Value=0
  Demux : Demux  Outputs=3
  Mux : Mux
  q(vect) : Outport
  wires:
  Vector [1 0 0]/1 -> Demux/1
  Mux/1 -> q(vect)/1
  Constant/1 -> Mux/4
  Demux/3 -> Mux/3
  Demux/2 -> Mux/2
  Demux/1 -> Mux/1

== system Dynamics_2024/Orbit Dynamics Perturbed/Spacecraft_Earth_J2 integrator /Subsystem4/Subsystem1 ==
  In1 : Inport
  Dot Product : DotProduct  OutDataTypeStr=Inherit: Inherit via internal rule
  Sqrt : Sqrt
  Out1 : Outport
  wires:
  Sqrt/1 -> Out1/1
  Dot Product/1 -> Sqrt/1
  In1/1 -> Dot Product/2, Dot Product/1

== system Dynamics_2024/attitude error/Attitude Error/Rotation of w_LN/Quaternion multiplication 1 ==
  q_BL' = q : Inport
  q_LN = q' : Inport  Port=2
  Demux : Demux
  Gain : Gain  Gain=[1 0 0 0; 0 1 0 0; 0 0 1 0; 0 0 0 1]
  Gain1 : Gain  Gain=[0 0 0 1; 0 0 1 0; 0 -1 0 0; -1 0 0 0]
  Gain2 : Gain  Gain=[0 0 -1 0; 0 0 0 1; 1 0 0 0; 0 -1 0 0]
  Gain3 : Gain  Gain=[0 1 0 0; -1 0 0 0; 0 0 0 1; 0 0 -1 0]
  Product : Product  Multiplication=Matrix(*)
  Sum : Sum  Inputs=|++++
  q*q' = q1 : Outport
  wires:
  q_LN = q'/1 -> Demux/1
  Demux/4 -> Gain/1
  Demux/1 -> Gain1/1
  Demux/2 -> Gain2/1
  Demux/3 -> Gain3/1
  Gain1/1 -> Sum/1
  Gain2/1 -> Sum/2
  Gain3/1 -> Sum/3
  Gain/1 -> Sum/4
  q_BL' = q/1 -> Product/2
  Sum/1 -> Product/1
  Product/1 -> q*q' = q1/1

== system Dynamics_2024/attitude error/Attitude Error/Rotation of w_LN/Quaternion multiplication 2 ==
  q1 = q : Inport
  q_BL = q' : Inport  Port=2
  Demux : Demux
  Gain : Gain  Gain=[1 0 0 0; 0 1 0 0; 0 0 1 0; 0 0 0 1]
  Gain1 : Gain  Gain=[0 0 0 1;0 0 1 0;0 -1 0 0;-1 0 0 0]
  Gain2 : Gain  Gain=[0 0 -1 0;0 0 0 1;1 0 0 0;0 -1 0 0]
  Gain3 : Gain  Gain=[0 1 0 0; -1 0 0 0; 0 0 0 1; 0 0 -1 0]
  Product : Product  Multiplication=Matrix(*)
  Sum : Sum  Inputs=|++++
  q*q' = q2 : Outport
  wires:
  q_BL = q'/1 -> Demux/1
  Demux/4 -> Gain/1
  Demux/1 -> Gain1/1
  Demux/2 -> Gain2/1
  Demux/3 -> Gain3/1
  Gain1/1 -> Sum/1
  Gain2/1 -> Sum/2
  Gain3/1 -> Sum/3
  Gain/1 -> Sum/4
  q1 = q/1 -> Product/2
  Sum/1 -> Product/1
  Product/1 -> q*q' = q2/1

== system Dynamics_2024/attitude error/Attitude Error/Rotation of w_LN/Transformation in Quaternion ==
  note: Adding 0 as fourth element
      | to match the Quaternion's dimension
  w_LN : Inport
  Constant : Constant  Value=0
  Demux : Demux  Outputs=3
  Mux : Mux
  q_LN : Outport
  wires:
  w_LN/1 -> Demux/1
  Mux/1 -> q_LN/1
  Constant/1 -> Mux/4
  Demux/3 -> Mux/3
  Demux/2 -> Mux/2
  Demux/1 -> Mux/1

== system Dynamics_2024/attitude error/Attitude Error/q_LN/Quaternion multiplication 1 ==
  q(om+theta) = q' : Inport
  q(i) = q : Inport  Port=2
  Demux : Demux
  Gain : Gain  Gain=[1 0 0 0; 0 1 0 0; 0 0 1 0; 0 0 0 1]
  Gain1 : Gain  Gain=[0 0 0 1; 0 0 1 0; 0 -1 0 0; -1 0 0 0]
  Gain2 : Gain  Gain=[0 0 -1 0; 0 0 0 1; 1 0 0 0; 0 -1 0 0]
  Gain3 : Gain  Gain=[0 1 0 0; -1 0 0 0; 0 0 0 1; 0 0 -1 0]
  Product : Product  Multiplication=Matrix(*)
  Sum : Sum  Inputs=|++++
  q*q' = q1 : Outport
  wires:
  q(om+theta) = q'/1 -> Demux/1
  Demux/4 -> Gain/1
  Demux/1 -> Gain1/1
  Demux/2 -> Gain2/1
  Demux/3 -> Gain3/1
  Gain1/1 -> Sum/1
  Gain2/1 -> Sum/2
  Gain3/1 -> Sum/3
  Gain/1 -> Sum/4
  q(i) = q/1 -> Product/2
  Sum/1 -> Product/1
  Product/1 -> q*q' = q1/1

== system Dynamics_2024/attitude error/Attitude Error/q_LN/Quaternion multiplication 2 ==
  q1 = q' : Inport
  q(OM) = q : Inport  Port=2
  Demux : Demux
  Gain : Gain  Gain=[1 0 0 0; 0 1 0 0; 0 0 1 0; 0 0 0 1]
  Gain1 : Gain  Gain=[0 0 0 1; 0 0 1 0; 0 -1 0 0; -1 0 0 0]
  Gain2 : Gain  Gain=[0 0 -1 0; 0 0 0 1; 1 0 0 0; 0 -1 0 0]
  Gain3 : Gain  Gain=[0 1 0 0; -1 0 0 0; 0 0 0 1; 0 0 -1 0]
  Product : Product  Multiplication=Matrix(*)
  Sum : Sum  Inputs=|++++
  q*q' = q2 : Outport
  wires:
  q1 = q'/1 -> Demux/1
  Demux/4 -> Gain/1
  Demux/1 -> Gain1/1
  Demux/2 -> Gain2/1
  Demux/3 -> Gain3/1
  Gain1/1 -> Sum/1
  Gain2/1 -> Sum/2
  Gain3/1 -> Sum/3
  Gain/1 -> Sum/4
  q(OM) = q/1 -> Product/2
  Sum/1 -> Product/1
  Product/1 -> q*q' = q2/1

== system Dynamics_2024/attitude error/Attitude Error/q_LN/Sign Determination1 ==
  "q_LN " : Inport
  q_BN : Inport  Port=2
  Function to determinate the correct sign of the estimated quaternion : MATLAB Function  TreatAsAtomicUnit=on
  Subsystem : Subsystem
  q_est : Outport
  wires:
  Subsystem/1(Out1) -> q_est/1
  "q_LN "/1 -> Function to determinate the correct sign of the estimated quaternion/2("q_est ")
  q_BN/1 -> Function to determinate the correct sign of the estimated quaternion/1(q_BN)
  Function to determinate the correct sign of the estimated quaternion/1(q_est) -> Subsystem/1(q_est)

== system Dynamics_2024/attitude error/Attitude Error/q_LN/Sign Determination1/Subsystem ==
  q_est : Inport
  Demux : Demux
  Mux : Mux
  Out1 : Outport
  wires:
  q_est/1 -> Demux/1
  Demux/1 -> Mux/1
  Demux/2 -> Mux/2
  Demux/3 -> Mux/3
  Demux/4 -> Mux/4
  Mux/1 -> Out1/1

== matlab function Dynamics_2024/Disturbances/MATLAB Function2 ==
  data: S_B input; M_SRP output; F_e input; A input; N_B input; R input
function M_SRP  = fcn(S_B, F_e,A,N_B,R)

c = 3e8;
M_SRP = [0; 0; 0];

rho_s = [0.5 0.1]';
rho_d = [0.1 0.1]';

P = F_e/c;
    for i = 1:length(N_B)
    N_Bi = N_B(:,i);
    DOT = dot(S_B,N_Bi); %[1x3][3x1] = [1x1]
    if DOT>0
        j = 1;
        if i>6
            j = 2;
        end
        F = -P*A(i)*DOT* ((1-rho_s(j))*S_B + (2*rho_s(j)*DOT+2/3*rho_d(j))*N_Bi);
        R_i = R(:,i);
        
        M_SRP = M_SRP + cross(R_i',F)'; 
    end
    end
end

== matlab function Dynamics_2024/Orbit Dynamics Perturbed/MATLAB Function ==
  data: r input; v input; inc output; omega output; w output; theta output
function [inc,omega,w,theta]=car2kep(r,v)
    
    mu=astroConstants(13);
    % norme di r e v
    mod_r=norm(r);
    mod_v=norm(v);
    
    % h
    h=cross(r,v);
    mod_h=norm(h);
    
    % inc
    inc=acos(h(3)/mod_h);
    
    % Energia 
    E=0.5*mod_v^2-mu/mod_r;
    a=-0.5*mu/E;
    
    % N
    if inc==0
        N=[1 0 0]';
        mod_N=1;
    else
    K=[0 0 1]';
    N=cross(K,h);
    mod_N=norm(N);
    end

    % e
    e=(1/mu)*(((mod_v^2-mu/mod_r)*r)-(dot(r,v)*v));
    mod_e=norm(e);

    if mod_e <= 1e-3
        e=N;
    end
    
    % omega
    if inc==0
        omega=0;
    elseif(N(2)>=0)
     omega=acos(N(1)/mod_N);
    else
     omega=2*pi-acos(N(1)/mod_N);   
    end
    
    % w
    if mod_e<=1e-3
        w=0;
    elseif(e(3)>=0)
        w=acos(dot(N,e)/(mod_e*mod_N));
    else
        w=2*pi-acos(dot(N,e)/(mod_e*mod_N));
    end
    
    % v_r
    v_r=dot(r,v)/mod_r;
    
    % theta
    if(v_r>=0)
     theta=acos(dot(e,r)/(mod_e*mod_r));
    else
     theta=2*pi-acos(dot(e,r)/(mod_e*mod_r));  
    end
    % bug nel caso di orbite circolari per determinare pi< theta < 2 pi

end

== matlab function Dynamics_2024/attitude error/Attitude Error/q_LN/Sign Determination1/Function to determinate the correct sign of the estimated quaternion ==
  data: q_BN input; q_est output; q_est input
function q_est = fcn(q_BN,q_est)

[~,index] = max(abs(q_BN));

if q_est(index)*q_BN(index)>0
    q_est = q_est;
else
    q_est = -q_est;
end
